simulink model "trajStiffLearning"  (R2014b)
settings: Solver=VariableStepAuto  StartTime=0.0  StopTime=T  RelTol=1e-3
values from neighbouring files (symbols this model uses):
  dt = dt_sim    (= 0.01)    [settings_ST.m]    (also in settings_ST_puma.m)
  dt_pilco = 0.1    [settings_ST.m]    (also in settings_ST_puma.m)
  dyno = [7 8 12 13 14 18 19]    [settings_ST.m]    (also in settings_ST_puma.m = [13 14 19 20 25 26])
  indices = 1:1:stateLength    [settings_ST.m]    (also in settings_ST_puma.m)
  initRollOutNoise = 1e-4    (= 0.0001)    [settings_ST.m]
  jj = J    [learnImp_ST.m]
  Kd_env = [200, 50, 0, 0, 0, 0]    [settings_ST.m]    (also in settings_ST_puma.m = [0, 0, 1, 0, 0, 0])
  Kp_env = [5e3, 1e3, 0, 0, 0, 0]    [settings_ST.m]    (also in settings_ST_puma.m = [1e4, 1e4, 1e4, 0, 0, 0])
  n = 3    [settings_ST.m]    (also in settings_ST_puma.m = robot.n)
  peg = 0    [settings_ST.m]    (also in settings_ST_puma.m)
  robot = p560    [settings_ST_puma.m]
  varTargets = [160, 160, 0, 0]    [settings_ST.m]
  xc = [0.45, 2, 2, 10, 10, 10]'    [settings_ST.m]    (also in settings_ST_puma.m = [0.45, 0.6, 0.6, 10, 10, 10]')
undefined symbols (not defined in the file or in its folder): addNoise, gaussian, jacob_dot, mu0, multTargets, plant, policy, random
libraries: roblocks x8, simulink x2
settings Model: Creator=victor  LastModifiedBy=LocalAdmin
settings DataIOCC: SaveFormat=Dataset
settings OptimizationCC: UseDivisionForNetSlopeComputation=off  SimCompilerOptimization=off
settings DebuggingCC: SolverPrmCheckMsg=none  FrameProcessingCompatibilityMsg=error  AllowSymbolicDim=off
settings HardwareCC: ProdBitPerPointer=64  ProdLargestAtomicFloat=Float  ProdIntDivRoundTo=Zero  ProdEndianess=LittleEndian  ProdWordSize=64  ProdHWDeviceType=Intel->x86-64 (Windows64)
settings RTWCC: RTWCompilerOptimization=off
settings GRTTargetCC: GeneratePreprocessorConditionals=Use local settings
settings ConfigComp: CovMetricSettings=dw  CovHtmlReporting=on  CovSaveCumulativeToWorkspaceVar=on  CovSaveSingleToWorkspaceVar=on  CovExternalEMLEnable=off

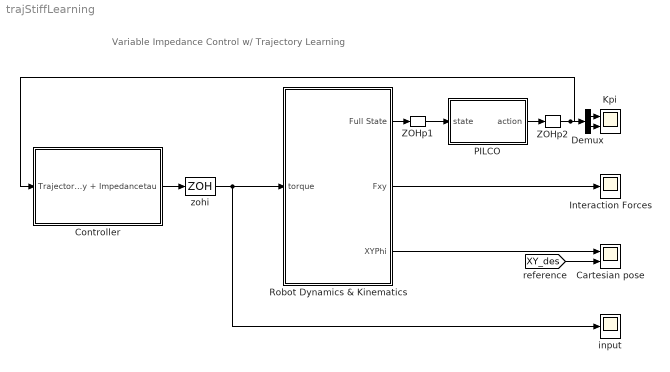
== system trajStiffLearning ==
  note: Variable Impedance Control w/ Trajectory Learning
  Cartesian pose : Scope  NumInputPorts=2
      settings: YMin=-0.11015~-5  YMax=0.56779~5
  Controller : Subsystem
  Demux : Demux  Outputs=2
  Interaction Forces : Scope
      settings: ShowLegends=on  YMin=-11.91054  YMax=75.21544  SaveName=ScopeData2
  Kpi : Scope  NumInputPorts=2
      settings: ShowLegends=on  YMin=10.68654~-0.05397  YMax=103.82157~-0.04029  SaveName=ScopeData3
  PILCO : Subsystem
  Robot Dynamics & Kinematics : Subsystem
  ZOHp1 : ZeroOrderHold  SampleTime=dt_pilco
  ZOHp2 : ZeroOrderHold  SampleTime=dt_pilco
  input : Scope
      settings: ShowLegends=on  YMin=-28.69807  YMax=16.88562  SaveName=ScopeData4
  zohi : ZeroOrderHold  SampleTime=dt
  wires:
  zohi/1 -> input/1, Robot Dynamics & Kinematics/1(torque)
  Controller/1(tau) -> zohi/1
  PILCO/1(action) -> ZOHp2/1
  Robot Dynamics & Kinematics/2(Fxy) -> Interaction Forces/1
  Robot Dynamics & Kinematics/1(Full State) -> ZOHp1/1
  Robot Dynamics & Kinematics/3(XYPhi) -> Cartesian pose/1
  [XY_des] -> Cartesian pose/2
  ZOHp1/1 -> PILCO/1(state)
  ZOHp2/1 -> Controller/1(Trajectory + Impedance), Demux/1
  Demux/1 -> Kpi/1
  Demux/2 -> Kpi/2

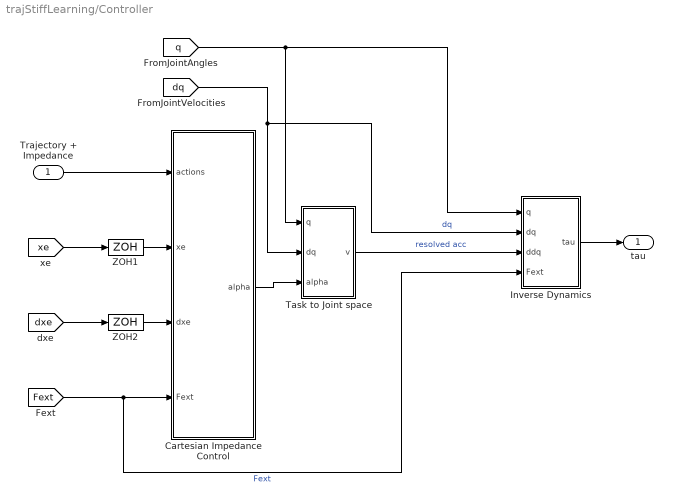
== system trajStiffLearning/Controller ==
  Trajectory + Impedance : Inport
  Cartesian Impedance Control : Subsystem
  Inverse Dynamics : Subsystem
  Task to Joint space : Subsystem
  ZOH1 : ZeroOrderHold  SampleTime=dt
  ZOH2 : ZeroOrderHold  SampleTime=dt
  tau : Outport
  wires:
  Cartesian Impedance Control/1(alpha) -> Task to Joint space/3(alpha)
  Task to Joint space/1(v) -> Inverse Dynamics/3(ddq)  "resolved acc"
  Inverse Dynamics/1(tau) -> tau/1
  [dq] -> Inverse Dynamics/2(dq), Task to Joint space/2(dq)  "dq"
  [Fext] -> Inverse Dynamics/4(Fext), Cartesian Impedance Control/4(Fext)  "Fext"
  Trajectory + Impedance/1 -> Cartesian Impedance Control/1(actions)
  [q] -> Task to Joint space/1(q), Inverse Dynamics/1(q)
  [xe] -> ZOH1/1
  [dxe] -> ZOH2/1
  ZOH1/1 -> Cartesian Impedance Control/2(xe)
  ZOH2/1 -> Cartesian Impedance Control/3(dxe)

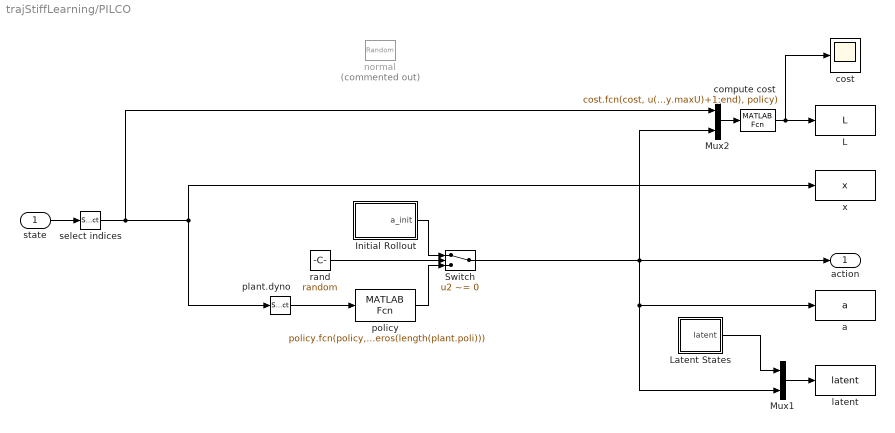
== system trajStiffLearning/PILCO ==
  state : Inport
  Initial Rollout : Subsystem
  L : ToWorkspace  VariableName=L  SampleTime=dt_pilco
  Latent States : Subsystem
  Mux1 : Mux  Inputs=2
  Mux2 : Mux  Inputs=2
  Switch : Switch  Criteria=u2 ~= 0
  a : ToWorkspace  VariableName=a  SampleTime=dt_pilco
  compute cost : MATLABFcn  MATLABFcn=cost.fcn(cost, u(plant.dyno), zeros(length(plant.dyno)), u(end-length(policy.maxU)+1:end), policy)  OutputDimensions=1  Output1D=off
  cost : Scope
      settings: ShowLegends=on  YMin=0.78643  YMax=1.02727  SaveName=L  SampleInput=on  SampleTime=dt_pilco
  latent : ToWorkspace  VariableName=latent  SampleTime=dt_pilco
  normal : RandomNumber  Commented=on  Mean=multTargets(jj,:)  Variance=varTargets  Seed=[1 2]  SampleTime=dt_pilco
  plant.dyno : Selector  InputPortWidth=length(indices)  Indices=plant.dyno
  policy : MATLABFcn  MATLABFcn=policy.fcn(policy, u(plant.poli), zeros(length(plant.poli)))
  rand : Constant  Value=random
  select indices : Selector  InputPortWidth=stateLength  Indices=indices
  x : ToWorkspace  VariableName=x  SampleTime=dt_pilco
  action : Outport
  wires:
  state/1 -> select indices/1
  Mux1/1 -> latent/1
  compute cost/1 -> cost/1, L/1
  plant.dyno/1 -> policy/1
  rand/1 -> Switch/2
  policy/1 -> Switch/3
  Initial Rollout/1(a_init) -> Switch/1
  Mux2/1 -> compute cost/1
  select indices/1 -> Mux2/1, x/1, plant.dyno/1
  Latent States/1(latent) -> Mux1/1
  Switch/1 -> action/1, a/1, Mux1/2, Mux2/2

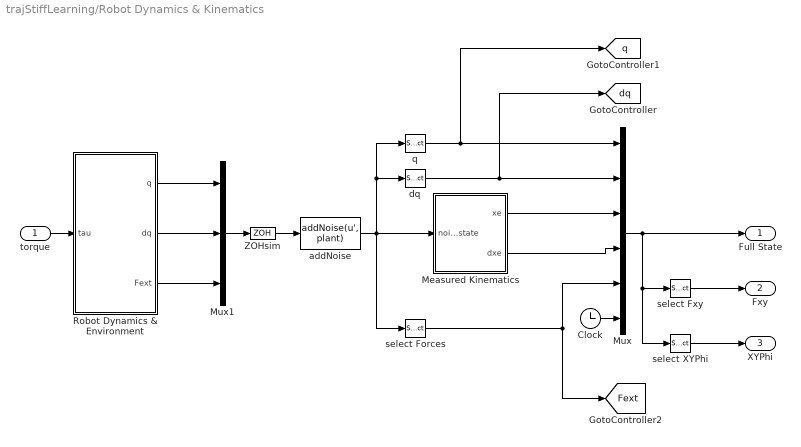
== system trajStiffLearning/Robot Dynamics & Kinematics ==
  torque : Inport
  Clock : Clock
  Measured Kinematics : Subsystem
  Mux : Mux  Inputs=6
  Mux1 : Mux  Inputs=3
  Robot Dynamics & Environment : Subsystem
  ZOHsim : ZeroOrderHold  SampleTime=dt
  addNoise : MATLABFcn  MATLABFcn=addNoise(u', plant)
  dq : Selector  InputPortWidth=2*robot.n+6  Indices=[robot.n+1:2*robot.n]
  q : Selector  InputPortWidth=2*robot.n+6  Indices=[1:robot.n]
  select Forces : Selector  InputPortWidth=2*robot.n+6  Indices=[2*robot.n+1:2*robot.n+6]
  select Fxy : Selector  InputPortWidth=stateLength  Indices=[19 20]
  select XYPhi : Selector  InputPortWidth=stateLength  Indices=[7 8 12]
  Full State : Outport
  Fxy : Outport  Port=2
  XYPhi : Outport  Port=3
  tag scope: Fext=global, dq=global, q=global
  wires:
  torque/1 -> Robot Dynamics & Environment/1(tau)
  Measured Kinematics/1(xe) -> Mux/3
  Measured Kinematics/2(dxe) -> Mux/4
  select Fxy/1 -> Fxy/1
  select XYPhi/1 -> XYPhi/1
  q/1 -> [q], Mux/1
  dq/1 -> [dq], Mux/2
  select Forces/1 -> Mux/5, [Fext]
  Robot Dynamics & Environment/1(q) -> Mux1/1
  Robot Dynamics & Environment/2(dq) -> Mux1/2
  Mux1/1 -> ZOHsim/1
  ZOHsim/1 -> addNoise/1
  addNoise/1 -> q/1, dq/1, select Forces/1, Measured Kinematics/1(noisy state)
  Robot Dynamics & Environment/3(Fext) -> Mux1/3
  Mux/1 -> Full State/1, select XYPhi/1, select Fxy/1
  Clock/1 -> Mux/6

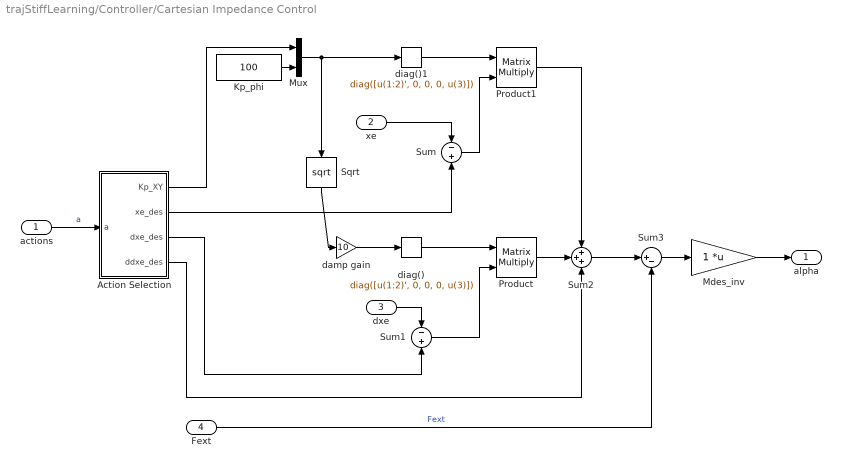
== system trajStiffLearning/Controller/Cartesian Impedance Control ==
  actions : Inport
  xe : Inport  Port=2
  dxe : Inport  Port=3
  Fext : Inport  Port=4
  Action Selection : Subsystem
  Kp_phi : Constant  Value=100
  Mdes_inv : Gain  Multiplication=Matrix(K*u)  SaturateOnIntegerOverflow=on  OutDataTypeStr=Inherit: Same as input  ParamDataTypeStr=Inherit: Same as input
  Mux : Mux  Inputs=2
  Product : Product  Multiplication=Matrix(*)
  Product1 : Product  Multiplication=Matrix(*)
  Sqrt : Sqrt  OutputSignalType=real  SaturateOnIntegerOverflow=on
  Sum : Sum  Inputs=-+  SaturateOnIntegerOverflow=on  InputSameDT=on  OutDataTypeStr=Inherit: Same as first input
  Sum1 : Sum  Inputs=-+  SaturateOnIntegerOverflow=on  InputSameDT=on  OutDataTypeStr=Inherit: Same as first input
  Sum2 : Sum  Inputs=+++  SaturateOnIntegerOverflow=on  InputSameDT=on  OutDataTypeStr=Inherit: Same as first input
  Sum3 : Sum  Inputs=|+-  SaturateOnIntegerOverflow=on  InputSameDT=on  OutDataTypeStr=Inherit: Same as first input
  damp gain : Gain  Gain=10  SaturateOnIntegerOverflow=on  OutDataTypeStr=Inherit: Same as input  ParamDataTypeStr=Inherit: Same as input
  diag() : MATLABFcn  MATLABFcn=diag([u(1:2)', 0, 0, 0, u(3)])  OutputDimensions=[6 6]  Output1D=off
  diag()1 : MATLABFcn  MATLABFcn=diag([u(1:2)', 0, 0, 0, u(3)])  OutputDimensions=[6 6]  Output1D=off
  alpha : Outport
  wires:
  Sum2/1 -> Sum3/1
  Sum3/1 -> Mdes_inv/1
  Action Selection/4(ddxe_des) -> Sum2/3
  Mdes_inv/1 -> alpha/1
  damp gain/1 -> diag()/1
  diag()/1 -> Product/1
  Mux/1 -> diag()1/1, Sqrt/1
  diag()1/1 -> Product1/1
  Sum/1 -> Product1/2
  Product1/1 -> Sum2/1
  Sum1/1 -> Product/2
  Product/1 -> Sum2/2
  Fext/1 -> Sum3/2  "Fext"
  Kp_phi/1 -> Mux/2
  Action Selection/2(xe_des) -> Sum/2
  actions/1 -> Action Selection/1(a)  "a"
  Action Selection/1(Kp_XY) -> Mux/1
  xe/1 -> Sum/1
  dxe/1 -> Sum1/1
  Action Selection/3(dxe_des) -> Sum1/2
  Sqrt/1 -> damp gain/1

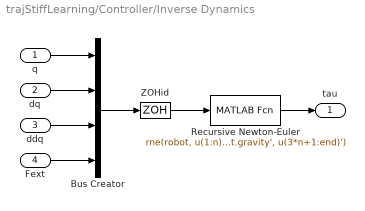
== system trajStiffLearning/Controller/Inverse Dynamics ==
  q : Inport
  dq : Inport  Port=2
  ddq : Inport  Port=3
  Fext : Inport  Port=4
  Bus Creator : BusCreator
  Recursive Newton-Euler : MATLABFcn  MATLABFcn=rne(robot, u(1:n)', u(n+1:2*n)', u(2*n+1:3*n)', robot.gravity', u(3*n+1:end)')  OutputDimensions=n
  ZOHid : ZeroOrderHold  SampleTime=dt
  tau : Outport
  wires:
  Recursive Newton-Euler/1 -> tau/1
  q/1 -> Bus Creator/1
  dq/1 -> Bus Creator/2
  ddq/1 -> Bus Creator/3
  Fext/1 -> Bus Creator/4
  Bus Creator/1 -> ZOHid/1
  ZOHid/1 -> Recursive Newton-Euler/1

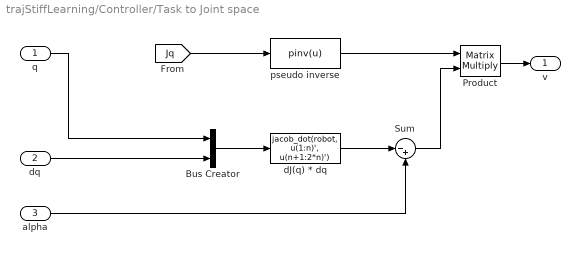
== system trajStiffLearning/Controller/Task to Joint space ==
  q : Inport
  dq : Inport  Port=2
  alpha : Inport  Port=3
  Bus Creator : BusCreator  Inputs=2
  Product : Product  Multiplication=Matrix(*)
  Sum : Sum  Inputs=|-+  SaturateOnIntegerOverflow=on  InputSameDT=on  OutDataTypeStr=Inherit: Same as first input
  dJ(q) * dq : MATLABFcn  MATLABFcn=jacob_dot(robot, u(1:n)', u(n+1:2*n)')  OutputDimensions=[6 1]  Output1D=off
  pseudo inverse : MATLABFcn  MATLABFcn=pinv(u)  Output1D=off
  v : Outport
  wires:
  [Jq] -> pseudo inverse/1
  dJ(q) * dq/1 -> Sum/1
  Sum/1 -> Product/2
  Product/1 -> v/1
  pseudo inverse/1 -> Product/1
  q/1 -> Bus Creator/1
  alpha/1 -> Sum/2
  dq/1 -> Bus Creator/2
  Bus Creator/1 -> dJ(q) * dq/1

== system trajStiffLearning/PILCO/Initial Rollout ==
  Initial Pos. References : FromWorkspace  VariableName=a_init{jj}  SampleTime=dt_pilco
  Initial Stiffness : FromWorkspace  VariableName=K0{jj}  SampleTime=dt_pilco
  Mux : Mux  Inputs=2
  XY_des : Selector  InputPortWidth=6  Indices=[1 2]
  a_init : Outport
  wires:
  Initial Pos. References/1 -> XY_des/1
  Initial Stiffness/1 -> Mux/1
  Mux/1 -> a_init/1
  XY_des/1 -> Mux/2

== system trajStiffLearning/PILCO/Latent States ==
  Mux : Mux  Inputs=5
  latent : Outport
  wires:
  [dq_latent] -> Mux/2
  [q_latent] -> Mux/1
  [Fext_latent] -> Mux/5
  [dxe_latent] -> Mux/4
  [xe_latent] -> Mux/3
  Mux/1 -> latent/1

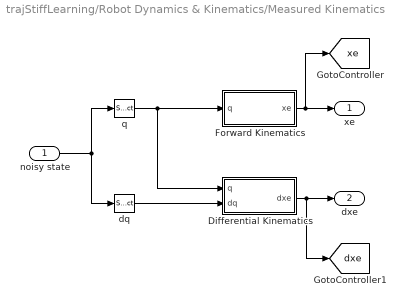
== system trajStiffLearning/Robot Dynamics & Kinematics/Measured Kinematics ==
  noisy state : Inport
  Differential Kinematics : Subsystem
  Forward Kinematics : Subsystem
  dq : Selector  InputPortWidth=2*robot.n + 6  Indices=[robot.n+1:2*robot.n]
  q : Selector  InputPortWidth=2*robot.n+6  Indices=[1:robot.n]
  xe : Outport
  dxe : Outport  Port=2
  tag scope: dxe=global, xe=global
  wires:
  Forward Kinematics/1(xe) -> [xe], xe/1
  q/1 -> Differential Kinematics/1(q), Forward Kinematics/1(q)
  noisy state/1 -> q/1, dq/1
  dq/1 -> Differential Kinematics/2(dq)
  Differential Kinematics/1(dxe) -> [dxe], dxe/1

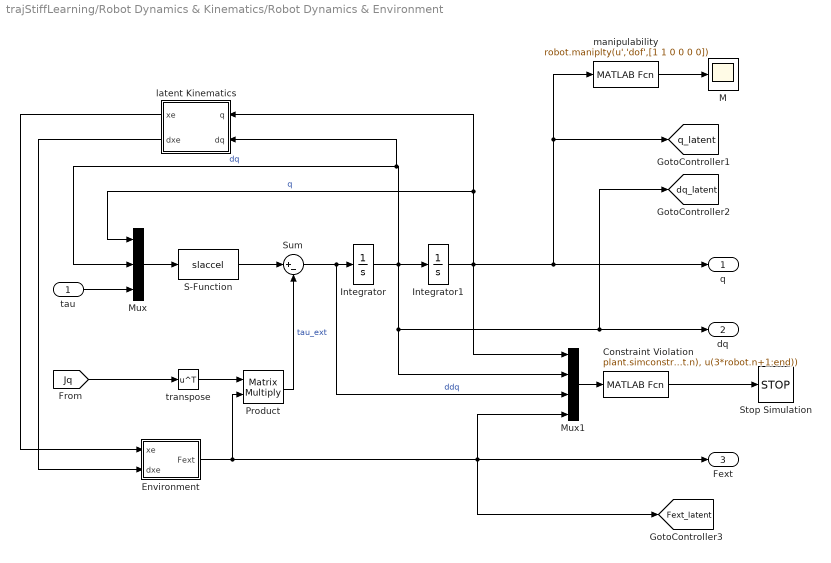
== system trajStiffLearning/Robot Dynamics & Kinematics/Robot Dynamics & Environment ==
  tau : Inport
  Constraint Violation : MATLABFcn  MATLABFcn=plant.simconstraint(u(1:robot.n), u(robot.n+1:2*robot.n), u(2*robot.n+1:3*robot.n), u(3*robot.n+1:end))
  Environment : Subsystem
  Integrator : Integrator
  Integrator1 : Integrator  InitialCondition=gaussian(mu0(1:robot.n),eye(robot.n)*initRollOutNoise,1)
  M : Scope
      settings: ShowLegends=on  YMin=0.13651  YMax=0.17434
  Mux : Mux  Inputs=3
  Mux1 : Mux
  Product : Product  Multiplication=Matrix(*)
  S-Function : S-Function  FunctionName=slaccel  Parameters=perturbedRobot  EnableBusSupport=off
  Stop Simulation : Stop
  Sum : Sum  Inputs=|+-
  latent Kinematics : Subsystem
  manipulability : MATLABFcn  MATLABFcn=robot.maniplty(u','dof',[1 1 0 0 0 0])
  transpose : Math  Operator=transpose  SaturateOnIntegerOverflow=on
  q : Outport
  dq : Outport  Port=2
  Fext : Outport  Port=3
  tag scope: Fext_latent=global, dq_latent=global, q_latent=global
  wires:
  S-Function/1 -> Sum/1
  Mux/1 -> S-Function/1
  Integrator/1 -> latent Kinematics/2(dq), Mux/2, Integrator1/1, Mux1/2, [dq_latent], dq/1  "dq"
  tau/1 -> Mux/3
  [Jq] -> transpose/1
  Product/1 -> Sum/2  "tau_ext"
  Integrator1/1 -> latent Kinematics/1(q), Mux/1, Mux1/1, q/1, manipulability/1, [q_latent]  "q"
  Sum/1 -> Mux1/3, Integrator/1  "ddq"
  transpose/1 -> Product/1
  Mux1/1 -> Constraint Violation/1
  Constraint Violation/1 -> Stop Simulation/1
  latent Kinematics/1(xe) -> Environment/1(xe)
  latent Kinematics/2(dxe) -> Environment/2(dxe)
  Environment/1(Fext) -> [Fext_latent], Fext/1, Mux1/4, Product/2
  manipulability/1 -> M/1

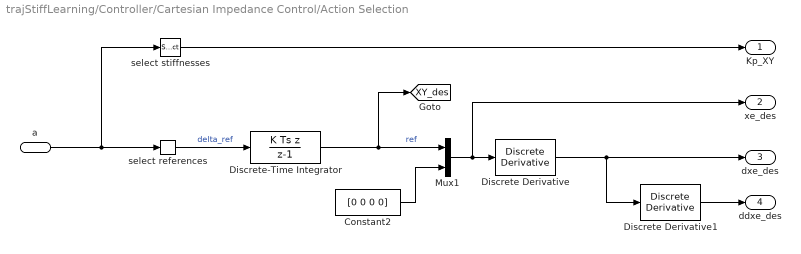
== system trajStiffLearning/Controller/Cartesian Impedance Control/Action Selection ==
  a : Inport
  Constant2 : Constant  Value=[0 0 0 0]
  Discrete Derivative : simulink/Discrete/Discrete Derivative  gainval=1.0  ICPrevScaledInput=0.0  InputProcessing=Inherited  OutMin=[]  OutMax=[]  OutDataType=fixdt(1, 16)  OutScaling=2^-10  DoSatur=off
  Discrete Derivative1 : simulink/Discrete/Discrete Derivative  gainval=1.0  ICPrevScaledInput=0.0  InputProcessing=Inherited  OutMin=[]  OutMax=[]  OutDataType=fixdt(1, 16)  OutScaling=2^-10  DoSatur=off
  Discrete-Time Integrator : DiscreteIntegrator  IntegratorMethod=Integration: Backward Euler  gainval=1/dt_pilco  InitialCondition=mu0(indices(dyno([1 2])))  InitialConditionSetting=State (most efficient)  SampleTime=dt_pilco  LimitOutput=on  UpperSaturationLimit=[0.6 0.5]  LowerSaturationLimit=[-0.6 -0.5]
  Mux1 : Mux  Inputs=2
  select references : Selector  InputPortWidth=length(policy.maxU)  Indices=policy.refIdx
  select stiffnesses : Selector  InputPortWidth=length(policy.maxU)  Indices=policy.impIdx
  Kp_XY : Outport
  xe_des : Outport  Port=2
  dxe_des : Outport  Port=3
  ddxe_des : Outport  Port=4
  tag scope: XY_des=global
  wires:
  a/1 -> select references/1, select stiffnesses/1
  Discrete Derivative/1 -> dxe_des/1, Discrete Derivative1/1
  select stiffnesses/1 -> Kp_XY/1
  Discrete Derivative1/1 -> ddxe_des/1
  Constant2/1 -> Mux1/2
  Mux1/1 -> Discrete Derivative/1, xe_des/1
  select references/1 -> Discrete-Time Integrator/1  "delta_ref"
  Discrete-Time Integrator/1 -> [XY_des], Mux1/1  "ref"

== system trajStiffLearning/Robot Dynamics & Kinematics/Measured Kinematics/Differential Kinematics ==
  q : Inport
  dq : Inport  Port=2
  Product : Product  Multiplication=Matrix(*)
  "jacob0 " : roblocks/Kinematics/jacob0 
  dxe : Outport
  wires:
  q/1 -> "jacob0 "/1
  Product/1 -> dxe/1  "dxe"
  dq/1 -> Product/2
  "jacob0 "/1 -> Product/1

== system trajStiffLearning/Robot Dynamics & Kinematics/Measured Kinematics/Forward Kinematics ==
  q : Inport
  Mux : Mux  Inputs=6
  T2rpy : roblocks/Transform Conversion/T2rpy
  T2xyz : roblocks/Transform Conversion/T2xyz
  fkine : roblocks/Kinematics/fkine
  xe : Outport
  wires:
  T2xyz/3 -> Mux/3  "z"
  T2rpy/3 -> Mux/6  "e"
  T2rpy/1 -> Mux/4  "a"
  T2xyz/2 -> Mux/2  "y"
  q/1 -> fkine/1
  fkine/1 -> T2rpy/1, T2xyz/1
  T2xyz/1 -> Mux/1  "x"
  T2rpy/2 -> Mux/5  "b"
  Mux/1 -> xe/1

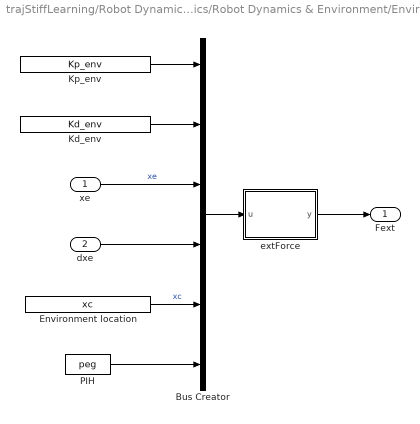
== system trajStiffLearning/Robot Dynamics & Kinematics/Robot Dynamics & Environment/Environment ==
  xe : Inport
  dxe : Inport  Port=2
  Bus Creator : BusCreator  Inputs=6
  Environment location : Constant  Value=xc  SampleTime=dt
  Kd_env : Constant  Value=Kd_env
  Kp_env : Constant  Value=Kp_env
  PIH : Constant  Value=peg  SampleTime=dt
  extForce : MATLAB Function  TreatAsAtomicUnit=on
  Fext : Outport
  wires:
  Environment location/1 -> Bus Creator/5  "xc"
  xe/1 -> Bus Creator/3  "xe"
  Bus Creator/1 -> extForce/1(u)
  Kp_env/1 -> Bus Creator/1
  Kd_env/1 -> Bus Creator/2
  dxe/1 -> Bus Creator/4
  extForce/1(y) -> Fext/1
  PIH/1 -> Bus Creator/6

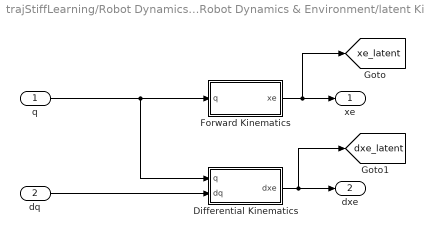
== system trajStiffLearning/Robot Dynamics & Kinematics/Robot Dynamics & Environment/latent Kinematics ==
  q : Inport
  dq : Inport  Port=2
  Differential Kinematics : Subsystem
  Forward Kinematics : Subsystem
  xe : Outport
  dxe : Outport  Port=2
  tag scope: dxe_latent=global, xe_latent=global
  wires:
  q/1 -> Differential Kinematics/1(q), Forward Kinematics/1(q)
  dq/1 -> Differential Kinematics/2(dq)
  Forward Kinematics/1(xe) -> [xe_latent], xe/1
  Differential Kinematics/1(dxe) -> [dxe_latent], dxe/1

== system trajStiffLearning/Robot Dynamics & Kinematics/Robot Dynamics & Environment/latent Kinematics/Differential Kinematics ==
  q : Inport
  dq : Inport  Port=2
  Product : Product  Multiplication=Matrix(*)
  "jacob0 " : roblocks/Kinematics/jacob0 
  dxe : Outport
  tag scope: Jq=global
  wires:
  q/1 -> "jacob0 "/1
  Product/1 -> dxe/1  "dxe"
  dq/1 -> Product/2
  "jacob0 "/1 -> Product/1, [Jq]

== system trajStiffLearning/Robot Dynamics & Kinematics/Robot Dynamics & Environment/latent Kinematics/Forward Kinematics ==
  q : Inport
  Mux : Mux  Inputs=6
  T2eul : roblocks/Transform Conversion/T2eul
  T2xyz : roblocks/Transform Conversion/T2xyz
  fkine : roblocks/Kinematics/fkine
  xe : Outport
  wires:
  T2xyz/3 -> Mux/3
  T2eul/3 -> Mux/6
  T2eul/1 -> Mux/4
  T2xyz/2 -> Mux/2
  q/1 -> fkine/1
  fkine/1 -> T2eul/1, T2xyz/1
  T2xyz/1 -> Mux/1
  T2eul/2 -> Mux/5
  Mux/1 -> xe/1

== matlab function trajStiffLearning/Robot Dynamics & Kinematics/Robot Dynamics & Environment/Environment/extForce ==
  data: u input; y output
function y = extForcefcn(u)
%Simulate external forces when performing PIH insertion.
% Environment is modelled as a spring+directional damping
%
% persistent inHole;
% 
% if isempty(inHole)
%     inHole =0;
% end

Fext = zeros(6,1);  %
Kp_env = u(1:6);    % environment stiffness
Kd_env = u(7:12);   % environment damping
xe = u(13:18);      % cartesian pose
dxe = u(19:24);     % cartesian velocity
xc = u(25:30);      % environment location
peg = u(31);        % PIH boolean
cf = 0.05;          % friction coefficient
insertStiffness = 75; % stiffness to overcome insertion.
contact = 0;
inHole = 0;

x_hole = [0.5, 0.1, 0];
r_hole = 0.005;          % tolerance per side of the peg

ywall_l = x_hole(2)+r_hole;
ywall_r = x_hole(2)-r_hole;

% determine state
if xe(1) > xc(1)
    contact = 1;
    if peg && xe(2) > ywall_r && xe(2) < ywall_l% && (xe(1) - xc(1)) > 0.01
        inHole = 1;
    end
end

if contact && ~inHole            % wall contact
    Fext(1) = Kp_env(1)*(xe(1)-xc(1));              % stiffness force -X
    if dxe(1) > 0
        Fext(1) = Fext(1) + Kd_env(1)*dxe(1);       % damping force   -X
    end
    
    Fext(2) = Fext(2) + cf * Fext(1) *-sign(dxe(2));% Coulomb friction +-Y
    
elseif contact && inHole    % peg is in hole
        
    if xe(1) > 0.48 && xe(1) < 0.52
        Fext(1) = insertStiffness*(xe(1) - 0.48);   % insertion resistance -X
    end
    
    if xe(1) > xc(1)+0.005
        %             Fext(1) = Kp_env(1)*(xe(1)-xc(1));              % stiffness force -X
        %             if xe(2) > ywall_l                              % wall stiffness -Y
        %                 Fext(2) = Kp_env(2)*(xe(2)-ywall_l);
        %             elseif xe(2) < ywall_r                          % wall stiffness +Y
        %                 Fext(2) = Kp_env(2)*(xe(2)-ywall_r);
        %             end
    end
end


% if Fext(1)>0  && isempty(inHole)                            % Frictional forces before insertion
%     Fext(2) = Fext(2) + cf * Fext(1) *-sign(dxe(2));
% end

y = Fext;
